simulink model "ESS5"  (R2017a)
settings: Solver=ode45  StartTime=0.0  StopTime=0.025  RelTol=1e-9
undefined symbols (not defined in the file): Delay_DF, Fs, OSR, Tau, Vmax, Vmin
libraries: dspmlti4 x5
settings Model: Creator=bhannigan  LastModifiedBy=bhannigan

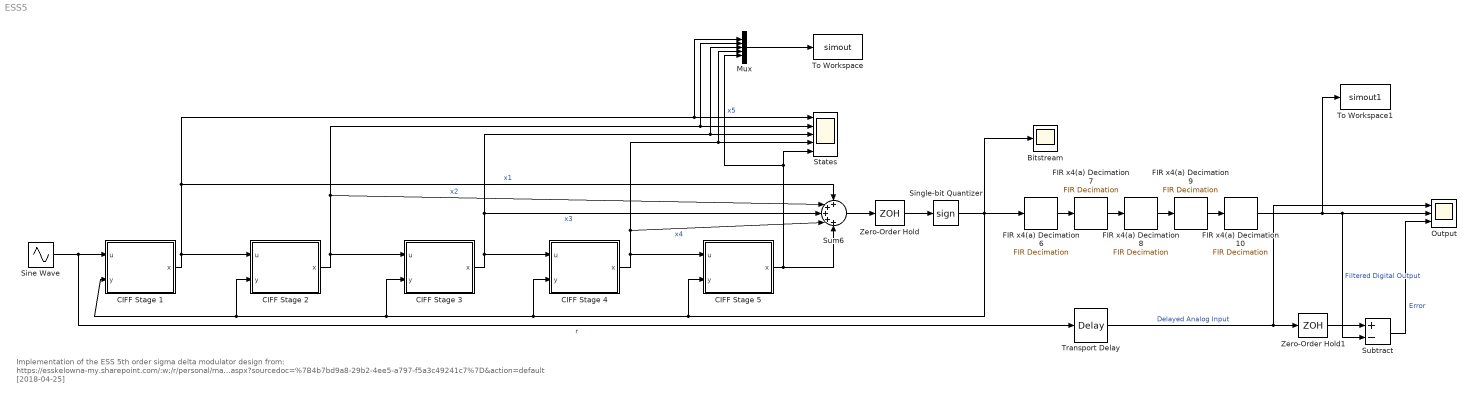
== system ESS5 ==
  note: Implementation of the ESS 5th order sigma delta modulator design from: https://esskelowna-my.sharepoint.com/:w:/r/personal/martin_esskelowna_onmicrosoft_com/_layouts/15/Doc.aspx?sourcedoc=%7B4b7bd9a8-29b2-4ee5-a797-f5a3c49241c7%7D&action=default [2018-04-25]
  Bitstream : Scope
  CIFF Stage 1 : Subsystem  mask(CIFF Stage){Tau=Tau(1), usat=Vmax(1), lsat=Vmin(1)}
      mask prompts: Tau "Time constant"; usat "Upper saturation limit"; lsat "Lower saturation limit"
      mask help: Clipped continuous-time integrator with variable time constant and feedforward output.
      mask DialogControl Container3 Prompt: test
  CIFF Stage 2 : Subsystem  mask(CIFF Stage){Tau=Tau(2), usat=Vmax(2), lsat=Vmin(2)}
      mask prompts: Tau "Time constant"; usat "Upper saturation limit"; lsat "Lower saturation limit"
      mask help: Clipped continuous-time integrator with variable time constant and feedforward output.
      mask DialogControl Container3 Prompt: test
  CIFF Stage 3 : Subsystem  mask(CIFF Stage){Tau=Tau(3), usat=Vmax(3), lsat=Vmin(3)}
      mask prompts: Tau "Time constant"; usat "Upper saturation limit"; lsat "Lower saturation limit"
      mask help: Clipped continuous-time integrator with variable time constant and feedforward output.
      mask DialogControl Container3 Prompt: test
  CIFF Stage 4 : Subsystem  mask(CIFF Stage){Tau=Tau(4), usat=Vmax(4), lsat=Vmin(4)}
      mask prompts: Tau "Time constant"; usat "Upper saturation limit"; lsat "Lower saturation limit"
      mask help: Clipped continuous-time integrator with variable time constant and feedforward output.
      mask DialogControl Container3 Prompt: test
  CIFF Stage 5 : Subsystem  mask(CIFF Stage){Tau=Tau(5), usat=Vmax(5), lsat=Vmin(5)}
      mask prompts: Tau "Time constant"; usat "Upper saturation limit"; lsat "Lower saturation limit"
      mask help: Clipped continuous-time integrator with variable time constant and feedforward output.
      mask DialogControl Container3 Prompt: test
  FIR x4(a) Decimation10 : dspmlti4/FIR Decimation  FilterSource=Dialog parameters  h=fir1(31,0.15)  D=4  filtStruct=Direct form  FilterObject=Hm_firdecim  framing=Allow multirate processing  inputOffset=0  outputBufInitCond=0  roundingMode=Floor  overflowMode=off  firstCoeffDataTypeStr=Inherit: Same word length as input  firstCoeffMin=[]  firstCoeffMax=[]  firstCoeffLastDataTypeStr=Inherit: Same word length as input  accumDataTypeStr=Inherit: Same as product output  accumLastDataTypeStr=Inherit: Same as product output  outputMin=[]  outputMax=[]
  FIR x4(a) Decimation{6..9} (4 alike) : dspmlti4/FIR Decimation  FilterSource=Dialog parameters  h=fir1(31,0.15)  D=2  filtStruct=Direct form  FilterObject=Hm_firdecim  framing=Allow multirate processing  inputOffset=0  outputBufInitCond=0  roundingMode=Floor  overflowMode=off  firstCoeffDataTypeStr=Inherit: Same word length as input  firstCoeffMin=[]  firstCoeffMax=[]  firstCoeffLastDataTypeStr=Inherit: Same word length as input  accumDataTypeStr=Inherit: Same as product output  accumLastDataTypeStr=Inherit: Same as product output  outputMin=[]  outputMax=[]
  Mux : Mux  Inputs=5
  Output : Scope  NumInputPorts=3
  Sine Wave : Sin  Amplitude=0.07  Frequency=2*pi*20000  SampleTime=0
  Single-bit Quantizer : Signum
  States : Scope  NumInputPorts=5
  Subtract : Sum  Inputs=+-
  Sum6 : Sum  Inputs=+++++
  To Workspace : ToWorkspace  VariableName=simout  SaveFormat=Timeseries  SampleTime=-1
  To Workspace1 : ToWorkspace  VariableName=simout1  SaveFormat=Timeseries  SampleTime=-1
  Transport Delay : TransportDelay  DelayTime=Delay_DF/Fs
  Zero-Order Hold : ZeroOrderHold  SampleTime=1/Fs
  Zero-Order Hold1 : ZeroOrderHold  SampleTime=OSR/Fs
  wires:
  Sum6/1 -> Zero-Order Hold/1
  Zero-Order Hold/1 -> Single-bit Quantizer/1
  FIR x4(a) Decimation6/1 -> FIR x4(a) Decimation7/1
  FIR x4(a) Decimation9/1 -> FIR x4(a) Decimation10/1
  FIR x4(a) Decimation8/1 -> FIR x4(a) Decimation9/1
  FIR x4(a) Decimation7/1 -> FIR x4(a) Decimation8/1
  FIR x4(a) Decimation10/1 -> To Workspace1/1, Output/2, Subtract/2  "Filtered Digital Output"
  CIFF Stage 1/1(x) -> CIFF Stage 2/1(u), Sum6/1, Mux/1, States/1  "x1"
  Sine Wave/1 -> Transport Delay/1, CIFF Stage 1/1(u)  "r"
  CIFF Stage 2/1(x) -> CIFF Stage 3/1(u), Sum6/2, Mux/2, States/2  "x2"
  Single-bit Quantizer/1 -> FIR x4(a) Decimation6/1, Bitstream/1, CIFF Stage 2/2(y), CIFF Stage 1/2(y), CIFF Stage 3/2(y), CIFF Stage 4/2(y), CIFF Stage 5/2(y)
  CIFF Stage 3/1(x) -> CIFF Stage 4/1(u), Sum6/3, Mux/3, States/3  "x3"
  CIFF Stage 4/1(x) -> CIFF Stage 5/1(u), Mux/4, States/4, Sum6/4  "x4"
  CIFF Stage 5/1(x) -> Sum6/5, Mux/5, States/5  "x5"
  Transport Delay/1 -> Output/1, Zero-Order Hold1/1  "Delayed Analog Input"
  Zero-Order Hold1/1 -> Subtract/1
  Subtract/1 -> Output/3  "Error"
  Mux/1 -> To Workspace/1

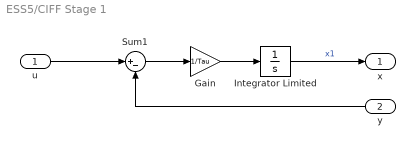
== system ESS5/CIFF Stage 1 ==
  u : Inport
  y : Inport  Port=2
  Gain : Gain  Gain=1/Tau
  Integrator Limited : Integrator  LimitOutput=on  UpperSaturationLimit=usat  LowerSaturationLimit=lsat  WrappedStateUpperValue=usat  WrappedStateLowerValue=lsat
  Sum1 : Sum  Inputs=|+-
  x : Outport
  wires:
  y/1 -> Sum1/2
  Sum1/1 -> Gain/1
  Integrator Limited/1 -> x/1  "x1"
  u/1 -> Sum1/1
  Gain/1 -> Integrator Limited/1

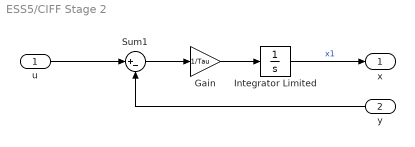
== system ESS5/CIFF Stage 2 ==
  u : Inport
  y : Inport  Port=2
  Gain : Gain  Gain=1/Tau
  Integrator Limited : Integrator  LimitOutput=on  UpperSaturationLimit=usat  LowerSaturationLimit=lsat  WrappedStateUpperValue=usat  WrappedStateLowerValue=lsat
  Sum1 : Sum  Inputs=|+-
  x : Outport
  wires:
  y/1 -> Sum1/2
  Sum1/1 -> Gain/1
  Integrator Limited/1 -> x/1  "x1"
  u/1 -> Sum1/1
  Gain/1 -> Integrator Limited/1

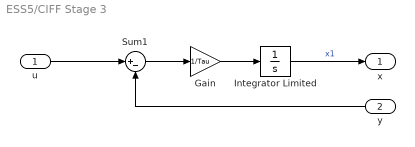
== system ESS5/CIFF Stage 3 ==
  u : Inport
  y : Inport  Port=2
  Gain : Gain  Gain=1/Tau
  Integrator Limited : Integrator  LimitOutput=on  UpperSaturationLimit=usat  LowerSaturationLimit=lsat  WrappedStateUpperValue=usat  WrappedStateLowerValue=lsat
  Sum1 : Sum  Inputs=|+-
  x : Outport
  wires:
  y/1 -> Sum1/2
  Sum1/1 -> Gain/1
  Integrator Limited/1 -> x/1  "x1"
  u/1 -> Sum1/1
  Gain/1 -> Integrator Limited/1

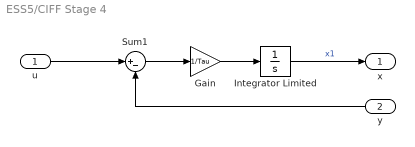
== system ESS5/CIFF Stage 4 ==
  u : Inport
  y : Inport  Port=2
  Gain : Gain  Gain=1/Tau
  Integrator Limited : Integrator  LimitOutput=on  UpperSaturationLimit=usat  LowerSaturationLimit=lsat  WrappedStateUpperValue=usat  WrappedStateLowerValue=lsat
  Sum1 : Sum  Inputs=|+-
  x : Outport
  wires:
  y/1 -> Sum1/2
  Sum1/1 -> Gain/1
  Integrator Limited/1 -> x/1  "x1"
  u/1 -> Sum1/1
  Gain/1 -> Integrator Limited/1

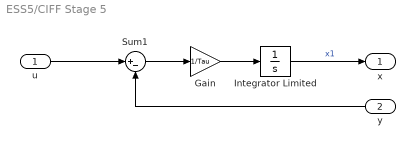
== system ESS5/CIFF Stage 5 ==
  u : Inport
  y : Inport  Port=2
  Gain : Gain  Gain=1/Tau
  Integrator Limited : Integrator  LimitOutput=on  UpperSaturationLimit=usat  LowerSaturationLimit=lsat  WrappedStateUpperValue=usat  WrappedStateLowerValue=lsat
  Sum1 : Sum  Inputs=|+-
  x : Outport
  wires:
  y/1 -> Sum1/2
  Sum1/1 -> Gain/1
  Integrator Limited/1 -> x/1  "x1"
  u/1 -> Sum1/1
  Gain/1 -> Integrator Limited/1
